simulink model "Simulink"  (R2023a)
settings: Solver=VariableStepAuto  StartTime=0.0  StopTime=2000/150e6  RelTol=1e-3
libraries: dspmlti4 x4
settings Model: Creator=Hasan  LastModifiedBy=Hasan
settings DataIOCC: ReturnWorkspaceOutputs=off
settings DebuggingCC: ParameterPrecisionLossMsg=none

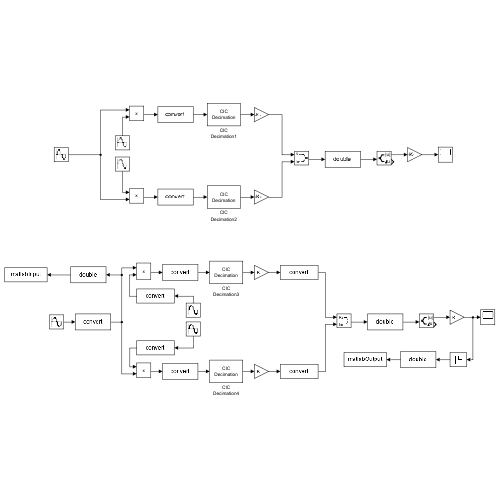
[thumbnail: Simulink's stored preview of the top-level diagram]
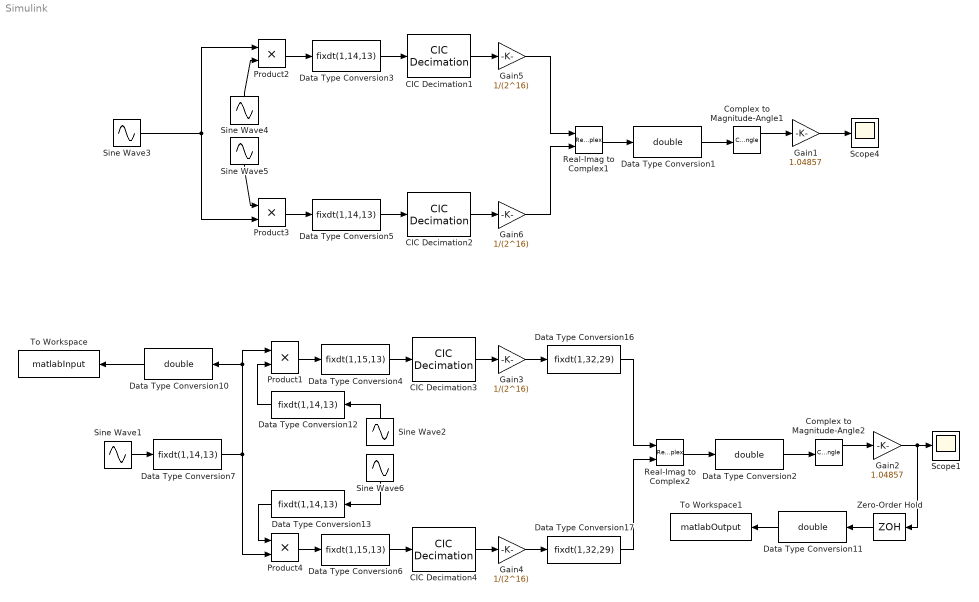
== system Simulink ==
  CIC Decimation1 : dspmlti4/CIC Decimation  filtFrom=Dialog parameters  filtobj=CICDECIM  ftype=Decimator  R=50  M=1  N=3  filterInternals=Full precision  BPS=[16 16 16 16]  FLPS=0  outputWordLength=50  outputFracLength=0  launchFVT=off  framing=Maintain input frame rate  RateOptions=Allow multirate processing
      settings: LibrarySourceBlock=|
      | dsphdlsupportfiltering/CIC
      | Decimation
  CIC Decimation2 : dspmlti4/CIC Decimation  filtFrom=Dialog parameters  filtobj=CICDECIM  ftype=Decimator  R=50  M=1  N=3  filterInternals=Full precision  BPS=[16 16 16 16]  FLPS=0  outputWordLength=50  outputFracLength=0  launchFVT=off  framing=Maintain input frame rate  RateOptions=Allow multirate processing
      settings: LibrarySourceBlock=|
      | dsphdlsupportfiltering/CIC
      | Decimation
  CIC Decimation3 : dspmlti4/CIC Decimation  filtFrom=Dialog parameters  filtobj=CICDECIM  ftype=Decimator  R=50  M=1  N=3  filterInternals=Full precision  BPS=[16 16 16 16]  FLPS=0  outputWordLength=14  outputFracLength=0  launchFVT=off  framing=Maintain input frame rate  RateOptions=Allow multirate processing
      settings: LibrarySourceBlock=|
      | dsphdlsupportfiltering/CIC
      | Decimation
  CIC Decimation4 : dspmlti4/CIC Decimation  filtFrom=Dialog parameters  filtobj=CICDECIM  ftype=Decimator  R=50  M=1  N=3  filterInternals=Full precision  BPS=[16 16 16 16]  FLPS=0  outputWordLength=50  outputFracLength=0  launchFVT=off  framing=Maintain input frame rate  RateOptions=Allow multirate processing
      settings: LibrarySourceBlock=|
      | dsphdlsupportfiltering/CIC
      | Decimation
  Complex to Magnitude-Angle1 : ComplexToMagnitudeAngle
  Complex to Magnitude-Angle2 : ComplexToMagnitudeAngle
  Data Type Conversion{1..2,10..11} (4 alike) : DataTypeConversion  OutDataTypeStr=double  SaturateOnIntegerOverflow=off  RndMeth=Floor
  Data Type Conversion{3,5,7,12..13} (5 alike) : DataTypeConversion  OutDataTypeStr=fixdt(1,14,13)  SaturateOnIntegerOverflow=off  RndMeth=Floor
  Data Type Conversion16 : DataTypeConversion  OutDataTypeStr=fixdt(1,32,29)  SaturateOnIntegerOverflow=off  RndMeth=Floor
  Data Type Conversion17 : DataTypeConversion  OutDataTypeStr=fixdt(1,32,29)  SaturateOnIntegerOverflow=off  RndMeth=Floor
  Data Type Conversion4 : DataTypeConversion  OutDataTypeStr=fixdt(1,15,13)  SaturateOnIntegerOverflow=off  RndMeth=Floor
  Data Type Conversion6 : DataTypeConversion  OutDataTypeStr=fixdt(1,15,13)  SaturateOnIntegerOverflow=off  RndMeth=Floor
  Gain1 : Gain  Gain=1.04857
  Gain2 : Gain  Gain=1.04857  ParamDataTypeStr=fixdt(1,14,12)  OutDataTypeStr=fixdt(1,45,41)
  Gain{3..6} (4 alike) : Gain  Gain=1/(2^16)
  Product{1..4} (4 alike) : Product
  Real-Imag to Complex1 : RealImagToComplex
  Real-Imag to Complex2 : RealImagToComplex
  Scope1 : Scope
  Scope4 : Scope
  Sine Wave1 : Sin  Frequency=2*pi*60e6  SampleTime=1/150e6
  Sine Wave2 : Sin  Frequency=2*pi*60e6  SampleTime=1/150e6
  Sine Wave3 : Sin  Frequency=2*pi*60e6  Phase=pi/4  SampleTime=1/150e6
  Sine Wave4 : Sin  Frequency=2*pi*60e6  SampleTime=1/150e6
  Sine Wave5 : Sin  Frequency=2*pi*60e6  Phase=pi/2  SampleTime=1/150e6
  Sine Wave6 : Sin  Frequency=2*pi*60e6  Phase=pi/2  SampleTime=1/150e6
  To Workspace : ToWorkspace  VariableName=matlabInput  SaveFormat=Timeseries  SampleTime=-1
  To Workspace1 : ToWorkspace  VariableName=matlabOutput  SaveFormat=Timeseries  SampleTime=-1
  Zero-Order Hold : ZeroOrderHold  SampleTime=1/150e6
  wires:
  Real-Imag to Complex1/1 -> Data Type Conversion1/1
  CIC Decimation1/1 -> Gain5/1
  Sine Wave5/1 -> Product3/1
  Sine Wave3/1 -> Product3/2, Product2/1
  Sine Wave4/1 -> Product2/2
  Product3/1 -> Data Type Conversion5/1
  Data Type Conversion3/1 -> CIC Decimation1/1
  Data Type Conversion5/1 -> CIC Decimation2/1
  CIC Decimation2/1 -> Gain6/1
  Data Type Conversion1/1 -> Complex to Magnitude-Angle1/1
  Complex to Magnitude-Angle1/1 -> Gain1/1
  Complex to Magnitude-Angle2/1 -> Gain2/1
  Data Type Conversion2/1 -> Complex to Magnitude-Angle2/1
  Data Type Conversion6/1 -> CIC Decimation4/1
  Data Type Conversion4/1 -> CIC Decimation3/1
  Product4/1 -> Data Type Conversion6/1
  Sine Wave1/1 -> Data Type Conversion7/1
  Sine Wave6/1 -> Data Type Conversion13/1
  Real-Imag to Complex2/1 -> Data Type Conversion2/1
  Data Type Conversion7/1 -> Data Type Conversion10/1, Product1/1, Product4/2
  Data Type Conversion10/1 -> To Workspace/1
  Data Type Conversion11/1 -> To Workspace1/1
  Gain2/1 -> Scope1/1, Zero-Order Hold/1
  Gain4/1 -> Data Type Conversion17/1
  Gain3/1 -> Data Type Conversion16/1
  Gain5/1 -> Real-Imag to Complex1/1
  Gain6/1 -> Real-Imag to Complex1/2
  Sine Wave2/1 -> Data Type Conversion12/1
  Data Type Conversion12/1 -> Product1/2
  Data Type Conversion13/1 -> Product4/1
  Data Type Conversion16/1 -> Real-Imag to Complex2/1
  Data Type Conversion17/1 -> Real-Imag to Complex2/2
  Product2/1 -> Data Type Conversion3/1
  Gain1/1 -> Scope4/1
  Zero-Order Hold/1 -> Data Type Conversion11/1
  CIC Decimation3/1 -> Gain3/1
  Product1/1 -> Data Type Conversion4/1
  CIC Decimation4/1 -> Gain4/1
